simulink model "testifintegratoriscorrect"  (R2019a)
settings: Solver=FixedStepAuto  StartTime=0.0  StopTime=100  FixedStep=1e-4  RelTol=1e-5
InitFcn:
  | HeightAboveSeaLevel = 400 * rand;
  | Temperature = 288.15 + 30 * (rand - 0.5);
  | Pressure = 	101325 + 6000 * (rand - 0.5);
  | 
  | GustStart = 5 * rand;
  | GustLength = [100 + 50 * (rand - 0.5), 100 + 50 * (rand - 0.5), 100 + 50 * (rand - 0.5)];
  | GuestAmplitude = [ 10 * (rand - 0.5), 10 * (rand - 0.5),  10 * (rand - 0.5)];
  | 
  | ShearSpeed = 20 * rand;
  | ShearDirection = 360 * rand;
  | 
  | HeightAboveSeaLevel = 5.4419142084;
  | Temperature = 288.15;
  | Pressure = 	101325;
  | 
  | GustStart = 2.5;
  | GustLength = [100, 100, 100];
  | GuestAmplitude = [ 2.5, -2.5,  1];
  | 
  | ShearSpeed = 10;
  | ShearDirection = 180;
values from neighbouring files (symbols this model uses):
  D = zeros(size(B))    [RocketOutputFunction.m]    (also in StateSpaceController.m = zeros(13, 3); TimeDelayCompensationElevator.m = [0; 0])
  F = eye(6)    [MEKFAttitudeOnly.m]
  Ki2 = lqr(Ai2, Bi2, Q, R)    [StateSpaceController.m]
  q = x(13:16)    [AdaptiveLQR.m]    (also in MEKF.m = nominal_state(4:7); MEKFAttitudeOnly.m = [1 0 0 0]; MEKF_old.m = nominal_state(4:7); NonlinearStateEstimationForActuatorDelay.m = x(4:7))
  r = sym('r', [3 1])    [StateSpaceController.m]    (also in TimeDelayCompensationElevator.m = [0;0]; Tracker.m = [0; 0; -(rocket_length - Average_cg)])
  s = linspace(0, 100, nums)    [ImpactVelocityFunction.m]    (also in ImpactVelocityNotParallelMatlab.m = 1:5:500; ParallelImpactVelocity.m = .1:.01:500; ParralelRun.m = linspace(5,7, nums); RunImpactVelocityParforCompiled.m = 1:0.1:500)
undefined symbols (not defined in the file or in its folder): deg, e0_0, e1_0, e2_0, e3_0, Earth, Light, magnitude, MIL, rad, WGS84
libraries: aerolibutil x10, simulink x9, aerolibconvert2 x7, sharedtransform x7, shared6dof x7, aerolibwind2 x3, sharedutil x3, aerolibfltsims x2, aerolibasang x2, shared6dofsys x2, aerolibatmos2 x1, aerolibbdyn x1
(part 1 of 2)
settings Model: Creator=rag  LastModifiedBy=rag
settings SolverCC: ZeroCrossAlgorithm=Adaptive  MinimalZcImpactIntegration=on
settings DataIOCC: SaveOutput=off  SignalLogging=off  DSMLogging=off  SaveTime=off
settings DebuggingCC: ReadBeforeWriteMsg=DisableAll  WriteAfterWriteMsg=DisableAll  WriteAfterReadMsg=DisableAll  IgnoredZcDiagnostic=none  MultiTaskDSMMsg=none
settings ModelReferenceCC: UpdateModelReferenceTargets=IfOutOfDate
settings SFSimCC: SFSimEcho=off

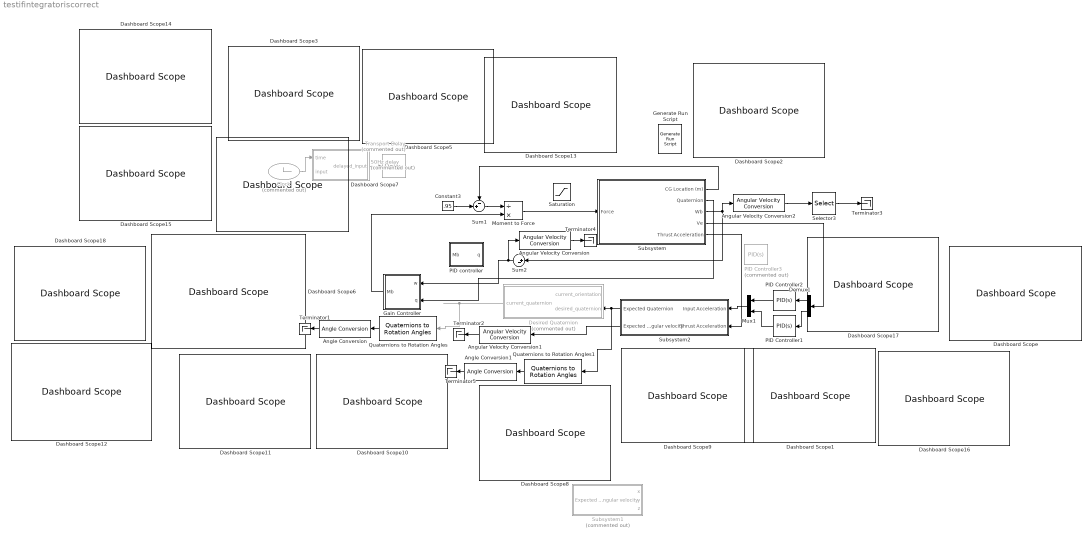
== system testifintegratoriscorrect ==
  50Hz delay : MATLAB Function  Commented=on  TreatAsAtomicUnit=on
  Angle Conversion : aerolibconvert2/Angle Conversion  IU=rad  OU=deg
  Angle Conversion1 : aerolibconvert2/Angle Conversion  IU=rad  OU=deg
  Angular Velocity Conversion : aerolibconvert2/Angular Velocity Conversion  IU=rad/s  OU=deg/s
      settings: SourceProductName=Aerospace Blockset
  Angular Velocity Conversion1 : aerolibconvert2/Angular Velocity Conversion  IU=rad/s  OU=deg/s
      settings: SourceProductName=Aerospace Blockset
  Angular Velocity Conversion2 : aerolibconvert2/Angular Velocity Conversion  IU=rad/s  OU=deg/s
      settings: SourceProductName=Aerospace Blockset
  Clock : Clock  Commented=on
      settings: Decimation=100
  Constant3 : Constant  Value=.95
  Dashboard Scope{,1..3,5..11,13..18} (17 alike) : DashboardScope
  Dashboard Scope12 : DashboardScope  Ymin=-1  Ymax=1
  Demux1 : Demux  Outputs=2
  Desired Quaternion : MATLAB Function  Commented=on  TreatAsAtomicUnit=on
  Gain Controller : Subsystem
  Generate Run Script : aerolibfltsims/Generate Run Script  Architecture=Win64  dataFlow=Send  GeometryModelName=Rocket  AirportId=PHNL  RunwayId=04L  InitialAltitude=13  InitialHeading=52.84  OffsetDistance=0  OffsetAzimuth=0  InstallScenery=off  DisableShaders=off  OriginAddress=127.0.0.1  DestinationPort=5502  OriginPort=5505  LocalAddress=127.0.0.1  OutputFileName=runfg.bat  FlightGearBaseDirectory=C:\Program Files\FlightGear 2018.2.2
  Moment to Force : Product  Inputs=/*
  Mux1 : Mux  Inputs=2
  PID Controller1 : simulink/Continuous/PID Controller  Controller=PID  Form=Parallel  TimeDomain=Continuous-time  SampleTime=-1  IntegratorMethod=Forward Euler  FilterMethod=Forward Euler  ControllerParametersSource=internal  P=-.5  I=-.5  D=0  UseFilter=on  N=10000  TunerSelectOption=Transfer Function Based (PID Tuner App)  InitialConditionSource=internal  InitialConditionForIntegrator=0  InitialConditionForFilter=0  DifferentiatorICPrevScaledInput=0  ExternalReset=none  TrackingMode=off  Kt=1  LimitOutput=off  UpperSaturationLimit=inf  LowerSaturationLimit=-inf  LinearizeAsGain=on  AntiWindupMode=none  Kb=1  POutMin=[]  POutMax=[]  IOutMin=[]  IOutMax=[]  DOutMin=[]  DOutMax=[]  NOutMin=[]  NOutMax=[]  SumOutMin=[]  SumOutMax=[]  SaturationOutMin=[]  SaturationOutMax=[]  PParamMin=[]  PParamMax=[]  IParamMin=[]  IParamMax=[]  DParamMin=[]  DParamMax=[]  NParamMin=[]  NParamMax=[]  KbParamMin=[]  KbParamMax=[]  KtParamMin=[]  KtParamMax=[]  KbOutMin=[]  KbOutMax=[]  KtOutMin=[]  KtOutMax=[]  IntegratorOutMin=[]  IntegratorOutMax=[]  FilterOutMin=[]  FilterOutMax=[]  SumI1OutMin=[]  SumI1OutMax=[]  SumI2OutMin=[]  SumI2OutMax=[]  SumI3OutMin=[]  SumI3OutMax=[]  SumI4OutMin=[]  SumI4OutMax=[]  SumDOutMin=[]  SumDOutMax=[]  DifferentiatorOutMin=[]  DifferentiatorOutMax=[]  FilterDiffOutCoefMin=[]  FilterDiffOutCoefMax=[]  ReciprocalOutMin=[]  ReciprocalOutMax=[]  SumDenOutMin=[]  SumDenOutMax=[]  SumNumOutMin=[]  SumNumOutMax=[]  DivideOutMin=[]  DivideOutMax=[]  IntegratorContinuousStateAttributes=''  IntegratorStateMustResolveToSignalObject=off  IntegratorRTWStateStorageClass=Auto  FilterContinuousStateAttributes=''  FilterStateMustResolveToSignalObject=off  FilterRTWStateStorageClass=Auto  ParallelPVariant=InternalParameters  IdealPVariant=Disabled  IVariant=InternalParameters  DVariant=InternalParameters  IntegratorVariant=Continuous  SatVariant=Disabled  AWVariant=Passthrough  PCopyVariant=Disabled  TRVariant=Disabled  FdbkBlocksVariant=Forward  IdealPFdbkVariant=Disabled  SatFdbkVariant=Disabled  DerivativeFilterVariant=ContFilter  NVariant=InternalParameters  NCopyVariant=Disabled  FilterICVariant=InternalICsFilter  IntegratorICVariant=InternalICs  ExternalResetVariant=Disabled  TRSumVariant=Passthrough  SumFdbkVariant=Disabled  SumVariant=Sum_PID
  PID Controller2 : simulink/Continuous/PID Controller  Controller=PID  Form=Parallel  TimeDomain=Continuous-time  SampleTime=-1  IntegratorMethod=Forward Euler  FilterMethod=Forward Euler  ControllerParametersSource=internal  P=-.5  I=-.5  D=0  UseFilter=on  N=10000  TunerSelectOption=Transfer Function Based (PID Tuner App)  InitialConditionSource=internal  InitialConditionForIntegrator=0  InitialConditionForFilter=0  DifferentiatorICPrevScaledInput=0  ExternalReset=none  TrackingMode=off  Kt=1  LimitOutput=off  UpperSaturationLimit=inf  LowerSaturationLimit=-inf  LinearizeAsGain=on  AntiWindupMode=none  Kb=1  POutMin=[]  POutMax=[]  IOutMin=[]  IOutMax=[]  DOutMin=[]  DOutMax=[]  NOutMin=[]  NOutMax=[]  SumOutMin=[]  SumOutMax=[]  SaturationOutMin=[]  SaturationOutMax=[]  PParamMin=[]  PParamMax=[]  IParamMin=[]  IParamMax=[]  DParamMin=[]  DParamMax=[]  NParamMin=[]  NParamMax=[]  KbParamMin=[]  KbParamMax=[]  KtParamMin=[]  KtParamMax=[]  KbOutMin=[]  KbOutMax=[]  KtOutMin=[]  KtOutMax=[]  IntegratorOutMin=[]  IntegratorOutMax=[]  FilterOutMin=[]  FilterOutMax=[]  SumI1OutMin=[]  SumI1OutMax=[]  SumI2OutMin=[]  SumI2OutMax=[]  SumI3OutMin=[]  SumI3OutMax=[]  SumI4OutMin=[]  SumI4OutMax=[]  SumDOutMin=[]  SumDOutMax=[]  DifferentiatorOutMin=[]  DifferentiatorOutMax=[]  FilterDiffOutCoefMin=[]  FilterDiffOutCoefMax=[]  ReciprocalOutMin=[]  ReciprocalOutMax=[]  SumDenOutMin=[]  SumDenOutMax=[]  SumNumOutMin=[]  SumNumOutMax=[]  DivideOutMin=[]  DivideOutMax=[]  IntegratorContinuousStateAttributes=''  IntegratorStateMustResolveToSignalObject=off  IntegratorRTWStateStorageClass=Auto  FilterContinuousStateAttributes=''  FilterStateMustResolveToSignalObject=off  FilterRTWStateStorageClass=Auto  ParallelPVariant=InternalParameters  IdealPVariant=Disabled  IVariant=InternalParameters  DVariant=InternalParameters  IntegratorVariant=Continuous  SatVariant=Disabled  AWVariant=Passthrough  PCopyVariant=Disabled  TRVariant=Disabled  FdbkBlocksVariant=Forward  IdealPFdbkVariant=Disabled  SatFdbkVariant=Disabled  DerivativeFilterVariant=ContFilter  NVariant=InternalParameters  NCopyVariant=Disabled  FilterICVariant=InternalICsFilter  IntegratorICVariant=InternalICs  ExternalResetVariant=Disabled  TRSumVariant=Passthrough  SumFdbkVariant=Disabled  SumVariant=Sum_PID
  PID Controller3 : simulink/Continuous/PID Controller  Commented=on  Controller=PID  Form=Parallel  TimeDomain=Continuous-time  SampleTime=-1  IntegratorMethod=Forward Euler  FilterMethod=Forward Euler  ControllerParametersSource=internal  P=-0.123834085166626  I=-0.0589771468563032  D=0.0137648749687481  UseFilter=on  N=8.99638285475018  TunerSelectOption=Transfer Function Based (PID Tuner App)  InitialConditionSource=internal  InitialConditionForIntegrator=0  InitialConditionForFilter=0  DifferentiatorICPrevScaledInput=0  ExternalReset=none  TrackingMode=off  Kt=1  LimitOutput=off  UpperSaturationLimit=inf  LowerSaturationLimit=-inf  LinearizeAsGain=on  AntiWindupMode=none  Kb=1  POutMin=[]  POutMax=[]  IOutMin=[]  IOutMax=[]  DOutMin=[]  DOutMax=[]  NOutMin=[]  NOutMax=[]  SumOutMin=[]  SumOutMax=[]  SaturationOutMin=[]  SaturationOutMax=[]  PParamMin=[]  PParamMax=[]  IParamMin=[]  IParamMax=[]  DParamMin=[]  DParamMax=[]  NParamMin=[]  NParamMax=[]  KbParamMin=[]  KbParamMax=[]  KtParamMin=[]  KtParamMax=[]  KbOutMin=[]  KbOutMax=[]  KtOutMin=[]  KtOutMax=[]  IntegratorOutMin=[]  IntegratorOutMax=[]  FilterOutMin=[]  FilterOutMax=[]  SumI1OutMin=[]  SumI1OutMax=[]  SumI2OutMin=[]  SumI2OutMax=[]  SumI3OutMin=[]  SumI3OutMax=[]  SumI4OutMin=[]  SumI4OutMax=[]  SumDOutMin=[]  SumDOutMax=[]  DifferentiatorOutMin=[]  DifferentiatorOutMax=[]  FilterDiffOutCoefMin=[]  FilterDiffOutCoefMax=[]  ReciprocalOutMin=[]  ReciprocalOutMax=[]  SumDenOutMin=[]  SumDenOutMax=[]  SumNumOutMin=[]  SumNumOutMax=[]  DivideOutMin=[]  DivideOutMax=[]  IntegratorContinuousStateAttributes=''  IntegratorStateMustResolveToSignalObject=off  IntegratorRTWStateStorageClass=Auto  FilterContinuousStateAttributes=''  FilterStateMustResolveToSignalObject=off  FilterRTWStateStorageClass=Auto  ParallelPVariant=InternalParameters  IdealPVariant=Disabled  IVariant=InternalParameters  DVariant=InternalParameters  IntegratorVariant=Continuous  SatVariant=Disabled  AWVariant=Passthrough  PCopyVariant=Disabled  TRVariant=Disabled  FdbkBlocksVariant=Forward  IdealPFdbkVariant=Disabled  SatFdbkVariant=Disabled  DerivativeFilterVariant=ContFilter  NVariant=InternalParameters  NCopyVariant=Disabled  FilterICVariant=InternalICsFilter  IntegratorICVariant=InternalICs  ExternalResetVariant=Disabled  TRSumVariant=Passthrough  SumFdbkVariant=Disabled  SumVariant=Sum_PID
  PID controller : Subsystem
  Quaternions to Rotation Angles : sharedtransform/Quaternions to Rotation Angles  rotationOrder=ZYX  aMode=aMode
      settings: SourceProductBaseCode=AE
  Quaternions to Rotation Angles1 : sharedtransform/Quaternions to Rotation Angles  rotationOrder=XYZ  aMode=aMode
      settings: SourceProductBaseCode=AE
  Saturation : Saturate  UpperLimit=1.5  LowerLimit=-1.5
  Selector3 : Selector  InputPortWidth=3  IndexOptions=Index vector (dialog)  Indices=[1 2]  OutputSizes=1
  Subsystem : Subsystem
  Subsystem1 : Subsystem  Commented=on
  Subsystem2 : Subsystem
  Sum1 : Sum  Inputs=-+|
  Sum2 : Sum  Inputs=|+-
  Terminator{1..5} (5 alike) : Terminator
  Transport Delay : TransportDelay  Commented=on  DelayTime=0.015  TransDelayFeedthrough=on
  wires:
  Subsystem/3(Wb) -> Sum2/1, Angular Velocity Conversion2/1
  Clock/1 -> 50Hz delay/1(time)
  50Hz delay/1(delayed_input) -> Transport Delay/1
  Sum2/1 -> Gain Controller/1(w), Angular Velocity Conversion/1
  Subsystem/5(Thrust Acceleration) -> Subsystem2/2(Thrust Acceleration)
  Angular Velocity Conversion1/1 -> Terminator2/1
  Subsystem2/2(Expected angular velocity) -> Angular Velocity Conversion1/1
  Quaternions to Rotation Angles/1 -> Angle Conversion/1
  Subsystem/1(CG Location (m)) -> Sum1/1
  Sum1/1 -> Moment to Force/1
  Constant3/1 -> Sum1/2
  Angle Conversion/1 -> Terminator1/1
  Angular Velocity Conversion2/1 -> Selector3/1
  Angular Velocity Conversion/1 -> Terminator4/1
  Angle Conversion1/1 -> Terminator5/1
  Subsystem2/1(Expected Quaternion) -> Desired Quaternion/2(desired_quaternion), Quaternions to Rotation Angles1/1
  Quaternions to Rotation Angles1/1 -> Angle Conversion1/1
  Desired Quaternion/1(current_quaternion) -> Quaternions to Rotation Angles/1
  Subsystem/2(Quaternion) -> Gain Controller/2(q)
  Gain Controller/1(Mb) -> Moment to Force/2
  Moment to Force/1 -> Subsystem/1(Force)
  Selector3/1 -> Terminator3/1
  Demux1/1 -> PID Controller2/1
  Mux1/1 -> Subsystem2/1(Input Acceleration)
  PID Controller2/1 -> Mux1/1
  Subsystem/4(Ve) -> Demux1/1
  Demux1/2 -> PID Controller1/1
  PID Controller1/1 -> Mux1/2

== system testifintegratoriscorrect/Gain Controller ==
  w : Inport
  q : Inport  Port=2
  Derivative : Derivative
  Gain : Gain  Gain=-Ki2  Multiplication=Matrix(K*u)
  Integrator : Integrator
  Reshape1 : Reshape  OutputDimensionality=Column vector (2-D)
  Selector1 : Selector  InputPortWidth=3  IndexOptions=Index vector (dialog)  Indices=[2 1]  OutputSizes=1
  Selector2 : Selector  InputPortWidth=4  IndexOptions=Index vector (dialog)  Indices=[3 2]  OutputSizes=1
  Vector Concatenate4 : Concatenate  NumInputs=3
  Mb : Outport
  wires:
  Vector Concatenate4/1 -> Reshape1/1
  Reshape1/1 -> Gain/1
  Selector2/1 -> Derivative/1, Integrator/1, Vector Concatenate4/2
  Integrator/1 -> Vector Concatenate4/3
  q/1 -> Selector2/1
  Gain/1 -> Mb/1
  Selector1/1 -> Vector Concatenate4/1
  w/1 -> Selector1/1

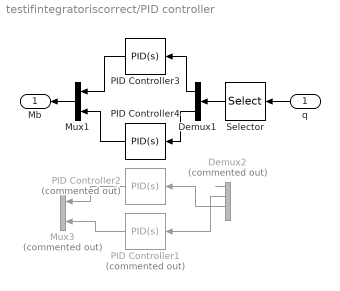
== system testifintegratoriscorrect/PID controller ==
  q : Inport
  Demux1 : Demux  Outputs=2
  Demux2 : Demux  Commented=on
  Mux1 : Mux  Inputs=2
  Mux3 : Mux  Commented=on  Inputs=2
  PID Controller1 : simulink/Continuous/PID Controller  Commented=on  Controller=PID  Form=Parallel  TimeDomain=Continuous-time  SampleTime=-1  IntegratorMethod=Forward Euler  FilterMethod=Forward Euler  ControllerParametersSource=internal  P=-19.0768820466686  I=-17.6802234864968  D=-5.0952523858048  UseFilter=on  N=209.794311620465  TunerSelectOption=Transfer Function Based (PID Tuner App)  InitialConditionSource=internal  InitialConditionForIntegrator=0  InitialConditionForFilter=0  DifferentiatorICPrevScaledInput=0  ExternalReset=none  TrackingMode=off  Kt=1  LimitOutput=off  UpperSaturationLimit=inf  LowerSaturationLimit=-inf  LinearizeAsGain=on  AntiWindupMode=none  Kb=1  POutMin=[]  POutMax=[]  IOutMin=[]  IOutMax=[]  DOutMin=[]  DOutMax=[]  NOutMin=[]  NOutMax=[]  SumOutMin=[]  SumOutMax=[]  SaturationOutMin=[]  SaturationOutMax=[]  PParamMin=[]  PParamMax=[]  IParamMin=[]  IParamMax=[]  DParamMin=[]  DParamMax=[]  NParamMin=[]  NParamMax=[]  KbParamMin=[]  KbParamMax=[]  KtParamMin=[]  KtParamMax=[]  KbOutMin=[]  KbOutMax=[]  KtOutMin=[]  KtOutMax=[]  IntegratorOutMin=[]  IntegratorOutMax=[]  FilterOutMin=[]  FilterOutMax=[]  SumI1OutMin=[]  SumI1OutMax=[]  SumI2OutMin=[]  SumI2OutMax=[]  SumI3OutMin=[]  SumI3OutMax=[]  SumI4OutMin=[]  SumI4OutMax=[]  SumDOutMin=[]  SumDOutMax=[]  DifferentiatorOutMin=[]  DifferentiatorOutMax=[]  FilterDiffOutCoefMin=[]  FilterDiffOutCoefMax=[]  ReciprocalOutMin=[]  ReciprocalOutMax=[]  SumDenOutMin=[]  SumDenOutMax=[]  SumNumOutMin=[]  SumNumOutMax=[]  DivideOutMin=[]  DivideOutMax=[]  IntegratorContinuousStateAttributes=''  IntegratorStateMustResolveToSignalObject=off  IntegratorRTWStateStorageClass=Auto  FilterContinuousStateAttributes=''  FilterStateMustResolveToSignalObject=off  FilterRTWStateStorageClass=Auto  ParallelPVariant=InternalParameters  IdealPVariant=Disabled  IVariant=InternalParameters  DVariant=InternalParameters  IntegratorVariant=Continuous  SatVariant=Disabled  AWVariant=Passthrough  PCopyVariant=Disabled  TRVariant=Disabled  FdbkBlocksVariant=Forward  IdealPFdbkVariant=Disabled  SatFdbkVariant=Disabled  DerivativeFilterVariant=ContFilter  NVariant=InternalParameters  NCopyVariant=Disabled  FilterICVariant=InternalICsFilter  IntegratorICVariant=InternalICs  ExternalResetVariant=Disabled  TRSumVariant=Passthrough  SumFdbkVariant=Disabled  SumVariant=Sum_PID
  PID Controller2 : simulink/Continuous/PID Controller  Commented=on  Controller=PID  Form=Parallel  TimeDomain=Continuous-time  SampleTime=-1  IntegratorMethod=Forward Euler  FilterMethod=Forward Euler  ControllerParametersSource=internal  P=-19.0768820466686  I=-17.6802234864968  D=-5.0952523858048  UseFilter=on  N=209.794311620465  TunerSelectOption=Transfer Function Based (PID Tuner App)  InitialConditionSource=internal  InitialConditionForIntegrator=0  InitialConditionForFilter=0  DifferentiatorICPrevScaledInput=0  ExternalReset=none  TrackingMode=off  Kt=1  LimitOutput=off  UpperSaturationLimit=inf  LowerSaturationLimit=-inf  LinearizeAsGain=on  AntiWindupMode=none  Kb=1  POutMin=[]  POutMax=[]  IOutMin=[]  IOutMax=[]  DOutMin=[]  DOutMax=[]  NOutMin=[]  NOutMax=[]  SumOutMin=[]  SumOutMax=[]  SaturationOutMin=[]  SaturationOutMax=[]  PParamMin=[]  PParamMax=[]  IParamMin=[]  IParamMax=[]  DParamMin=[]  DParamMax=[]  NParamMin=[]  NParamMax=[]  KbParamMin=[]  KbParamMax=[]  KtParamMin=[]  KtParamMax=[]  KbOutMin=[]  KbOutMax=[]  KtOutMin=[]  KtOutMax=[]  IntegratorOutMin=[]  IntegratorOutMax=[]  FilterOutMin=[]  FilterOutMax=[]  SumI1OutMin=[]  SumI1OutMax=[]  SumI2OutMin=[]  SumI2OutMax=[]  SumI3OutMin=[]  SumI3OutMax=[]  SumI4OutMin=[]  SumI4OutMax=[]  SumDOutMin=[]  SumDOutMax=[]  DifferentiatorOutMin=[]  DifferentiatorOutMax=[]  FilterDiffOutCoefMin=[]  FilterDiffOutCoefMax=[]  ReciprocalOutMin=[]  ReciprocalOutMax=[]  SumDenOutMin=[]  SumDenOutMax=[]  SumNumOutMin=[]  SumNumOutMax=[]  DivideOutMin=[]  DivideOutMax=[]  IntegratorContinuousStateAttributes=''  IntegratorStateMustResolveToSignalObject=off  IntegratorRTWStateStorageClass=Auto  FilterContinuousStateAttributes=''  FilterStateMustResolveToSignalObject=off  FilterRTWStateStorageClass=Auto  ParallelPVariant=InternalParameters  IdealPVariant=Disabled  IVariant=InternalParameters  DVariant=InternalParameters  IntegratorVariant=Continuous  SatVariant=Disabled  AWVariant=Passthrough  PCopyVariant=Disabled  TRVariant=Disabled  FdbkBlocksVariant=Forward  IdealPFdbkVariant=Disabled  SatFdbkVariant=Disabled  DerivativeFilterVariant=ContFilter  NVariant=InternalParameters  NCopyVariant=Disabled  FilterICVariant=InternalICsFilter  IntegratorICVariant=InternalICs  ExternalResetVariant=Disabled  TRSumVariant=Passthrough  SumFdbkVariant=Disabled  SumVariant=Sum_PID
  PID Controller3 : simulink/Continuous/PID Controller  Controller=PID  Form=Parallel  TimeDomain=Continuous-time  SampleTime=-1  IntegratorMethod=Forward Euler  FilterMethod=Forward Euler  ControllerParametersSource=internal  P=-19.0768820466686  I=-17.6802234864968  D=-5.0952523858048  UseFilter=on  N=209.794311620465  TunerSelectOption=Transfer Function Based (PID Tuner App)  InitialConditionSource=internal  InitialConditionForIntegrator=0  InitialConditionForFilter=0  DifferentiatorICPrevScaledInput=0  ExternalReset=none  TrackingMode=off  Kt=1  LimitOutput=off  UpperSaturationLimit=inf  LowerSaturationLimit=-inf  LinearizeAsGain=on  AntiWindupMode=none  Kb=1  POutMin=[]  POutMax=[]  IOutMin=[]  IOutMax=[]  DOutMin=[]  DOutMax=[]  NOutMin=[]  NOutMax=[]  SumOutMin=[]  SumOutMax=[]  SaturationOutMin=[]  SaturationOutMax=[]  PParamMin=[]  PParamMax=[]  IParamMin=[]  IParamMax=[]  DParamMin=[]  DParamMax=[]  NParamMin=[]  NParamMax=[]  KbParamMin=[]  KbParamMax=[]  KtParamMin=[]  KtParamMax=[]  KbOutMin=[]  KbOutMax=[]  KtOutMin=[]  KtOutMax=[]  IntegratorOutMin=[]  IntegratorOutMax=[]  FilterOutMin=[]  FilterOutMax=[]  SumI1OutMin=[]  SumI1OutMax=[]  SumI2OutMin=[]  SumI2OutMax=[]  SumI3OutMin=[]  SumI3OutMax=[]  SumI4OutMin=[]  SumI4OutMax=[]  SumDOutMin=[]  SumDOutMax=[]  DifferentiatorOutMin=[]  DifferentiatorOutMax=[]  FilterDiffOutCoefMin=[]  FilterDiffOutCoefMax=[]  ReciprocalOutMin=[]  ReciprocalOutMax=[]  SumDenOutMin=[]  SumDenOutMax=[]  SumNumOutMin=[]  SumNumOutMax=[]  DivideOutMin=[]  DivideOutMax=[]  IntegratorContinuousStateAttributes=''  IntegratorStateMustResolveToSignalObject=off  IntegratorRTWStateStorageClass=Auto  FilterContinuousStateAttributes=''  FilterStateMustResolveToSignalObject=off  FilterRTWStateStorageClass=Auto  ParallelPVariant=InternalParameters  IdealPVariant=Disabled  IVariant=InternalParameters  DVariant=InternalParameters  IntegratorVariant=Continuous  SatVariant=Disabled  AWVariant=Passthrough  PCopyVariant=Disabled  TRVariant=Disabled  FdbkBlocksVariant=Forward  IdealPFdbkVariant=Disabled  SatFdbkVariant=Disabled  DerivativeFilterVariant=ContFilter  NVariant=InternalParameters  NCopyVariant=Disabled  FilterICVariant=InternalICsFilter  IntegratorICVariant=InternalICs  ExternalResetVariant=Disabled  TRSumVariant=Passthrough  SumFdbkVariant=Disabled  SumVariant=Sum_PID
  PID Controller4 : simulink/Continuous/PID Controller  Controller=PID  Form=Parallel  TimeDomain=Continuous-time  SampleTime=-1  IntegratorMethod=Forward Euler  FilterMethod=Forward Euler  ControllerParametersSource=internal  P=-19.0768820466686  I=-17.6802234864968  D=-5.0952523858048  UseFilter=on  N=209.794311620465  TunerSelectOption=Transfer Function Based (PID Tuner App)  InitialConditionSource=internal  InitialConditionForIntegrator=0  InitialConditionForFilter=0  DifferentiatorICPrevScaledInput=0  ExternalReset=none  TrackingMode=off  Kt=1  LimitOutput=off  UpperSaturationLimit=inf  LowerSaturationLimit=-inf  LinearizeAsGain=on  AntiWindupMode=none  Kb=1  POutMin=[]  POutMax=[]  IOutMin=[]  IOutMax=[]  DOutMin=[]  DOutMax=[]  NOutMin=[]  NOutMax=[]  SumOutMin=[]  SumOutMax=[]  SaturationOutMin=[]  SaturationOutMax=[]  PParamMin=[]  PParamMax=[]  IParamMin=[]  IParamMax=[]  DParamMin=[]  DParamMax=[]  NParamMin=[]  NParamMax=[]  KbParamMin=[]  KbParamMax=[]  KtParamMin=[]  KtParamMax=[]  KbOutMin=[]  KbOutMax=[]  KtOutMin=[]  KtOutMax=[]  IntegratorOutMin=[]  IntegratorOutMax=[]  FilterOutMin=[]  FilterOutMax=[]  SumI1OutMin=[]  SumI1OutMax=[]  SumI2OutMin=[]  SumI2OutMax=[]  SumI3OutMin=[]  SumI3OutMax=[]  SumI4OutMin=[]  SumI4OutMax=[]  SumDOutMin=[]  SumDOutMax=[]  DifferentiatorOutMin=[]  DifferentiatorOutMax=[]  FilterDiffOutCoefMin=[]  FilterDiffOutCoefMax=[]  ReciprocalOutMin=[]  ReciprocalOutMax=[]  SumDenOutMin=[]  SumDenOutMax=[]  SumNumOutMin=[]  SumNumOutMax=[]  DivideOutMin=[]  DivideOutMax=[]  IntegratorContinuousStateAttributes=''  IntegratorStateMustResolveToSignalObject=off  IntegratorRTWStateStorageClass=Auto  FilterContinuousStateAttributes=''  FilterStateMustResolveToSignalObject=off  FilterRTWStateStorageClass=Auto  ParallelPVariant=InternalParameters  IdealPVariant=Disabled  IVariant=InternalParameters  DVariant=InternalParameters  IntegratorVariant=Continuous  SatVariant=Disabled  AWVariant=Passthrough  PCopyVariant=Disabled  TRVariant=Disabled  FdbkBlocksVariant=Forward  IdealPFdbkVariant=Disabled  SatFdbkVariant=Disabled  DerivativeFilterVariant=ContFilter  NVariant=InternalParameters  NCopyVariant=Disabled  FilterICVariant=InternalICsFilter  IntegratorICVariant=InternalICs  ExternalResetVariant=Disabled  TRSumVariant=Passthrough  SumFdbkVariant=Disabled  SumVariant=Sum_PID
  Selector : Selector  InputPortWidth=4  IndexOptions=Index vector (dialog)  Indices=[3 2]  OutputSizes=1
  Mb : Outport
  wires:
  q/1 -> Selector/1
  PID Controller1/1 -> Mux3/2
  Demux2/3 -> PID Controller2/1
  PID Controller2/1 -> Mux3/1
  Demux2/2 -> PID Controller1/1
  Demux2/1 -> ?
  Selector/1 -> Demux1/1
  PID Controller3/1 -> Mux1/1
  Demux1/1 -> PID Controller3/1
  Demux1/2 -> PID Controller4/1
  PID Controller4/1 -> Mux1/2
  Mux1/1 -> Mb/1

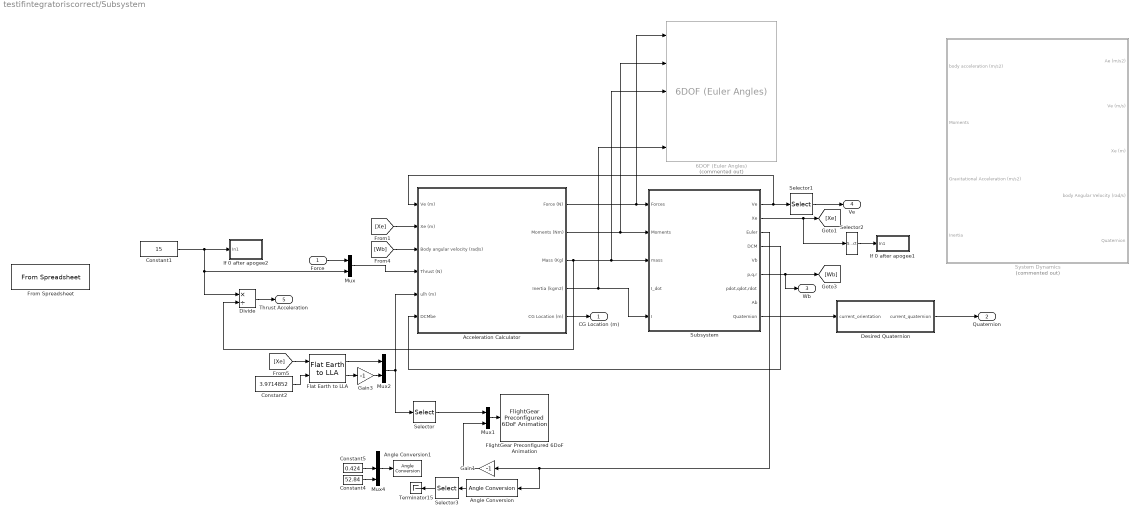
== system testifintegratoriscorrect/Subsystem ==
  Force : Inport  PortDimensions=2
  6DOF (Euler Angles) : shared6dof/6DOF (Euler Angles)  Commented=on  units=Metric (MKS)  mtype=Custom Variable  rep=Quaternion  xme_0=[0 0 0]  Vm_0=[0 0 0]  eul_0=[0 0 0]  pm_0=[0 0 0]  mass_0=1.0  mass_e=0.5  mass_f=2.0  inertia=eye(3)  inertia_e=eye(3)  inertia_f=2*eye(3)  k_quat=1.0  vre_flag=off  abi_flag=off  aMode=0  xme_statename=''  Vm_statename=''  eul_statename=''  quat_statename=''  pm_statename=''  mass_statename=''
      settings: SourceProductBaseCode=AE
  Acceleration Calculator : Subsystem
  Angle Conversion : aerolibconvert2/Angle Conversion  IU=rad  OU=deg
  Angle Conversion1 : aerolibconvert2/Angle Conversion  IU=deg  OU=rad
  Constant1 : Constant  Value=15
  Constant2 : Constant  Value=3.9714852
  Constant4 : Constant  Value=52.84
  Constant5 : Constant  Value=0.424
  Desired Quaternion : MATLAB Function  TreatAsAtomicUnit=on
  Divide : Product  Inputs=*/
  Flat Earth to LLA : aerolibtransform2/Flat Earth to LLA  units=Metric (MKS)  ptype=Earth (WGS84)  F=1/298.257223563  R=6378137  LL0=[21.318358277648 -157.9232805920725]  psi=0
  FlightGear Preconfigured 6DoF Animation : aerolibfltsims/FlightGear Preconfigured 6DoF Animation  xFlightGearVersion=v2018.2  DestinationIpAddress=127.0.0.1  DestinationPort=5502  SampleTime=1/50  packetVersion=24
      settings: SourceProductName=Aerospace Blockset
  From Spreadsheet : FromSpreadsheet  FileName=F10_Thrust.xls  Range=A1:B29  ExtrapolationBeforeFirstDataPoint=Hold first value  ExtrapolationAfterLastDataPoint=Hold last value
  Gain1 : Gain  Gain=-1
  Gain3 : Gain  Gain=-1
  If 0 after apogee1 : Subsystem
  If 0 after apogee2 : Subsystem
  Mux : Mux  Inputs=2
  Mux1 : Mux  Inputs=2
  Mux2 : Mux  Inputs=2
  Mux4 : Mux  Inputs=3
  Selector : Selector  InputPortWidth=3  IndexOptions=Index vector (dialog)  Indices=[2 1 3]  OutputSizes=1
  Selector1 : Selector  InputPortWidth=3  IndexOptions=Index vector (dialog)  Indices=[1 2]  OutputSizes=1
  Selector2 : Selector  InputPortWidth=3  IndexOptions=Index vector (dialog)  Indices=[3]  OutputSizes=1
  Selector3 : Selector  InputPortWidth=3  IndexOptions=Index vector (dialog)  Indices=[1 2]  OutputSizes=1
  Subsystem : Subsystem
  System Dynamics : Subsystem  Commented=on
  Terminator15 : Terminator
  CG Location (m) : Outport
  Quaternion : Outport  Port=2
  Wb : Outport  Port=3
  Ve : Outport  Port=4
  Thrust Acceleration : Outport  Port=5
  wires:
  Selector/1 -> Mux1/1
  Flat Earth to LLA/1 -> Mux2/1
  Flat Earth to LLA/2 -> Gain3/1
  Gain3/1 -> Mux2/2
  Mux2/1 -> Acceleration Calculator/5(ulh (m)), Selector/1
  Constant2/1 -> Flat Earth to LLA/2
  Subsystem/1(Ve) -> Acceleration Calculator/1(Ve (m)), Selector1/1
  Mux1/1 -> FlightGear Preconfigured 6DoF Animation/1
  [Xe] -> Acceleration Calculator/2(Xe (m))
  Force/1 -> Mux/1
  Selector2/1 -> If 0 after apogee1/1(In1)
  Constant4/1 -> Mux4/3
  Mux4/1 -> Angle Conversion1/1
  Constant5/1 -> Mux4/2
  [Xe] -> Flat Earth to LLA/1
  Divide/1 -> Thrust Acceleration/1
  [Wb] -> Acceleration Calculator/3(Body angular velocity (rad/s))
  Acceleration Calculator/5(CG Location (m)) -> CG Location (m)/1
  Selector1/1 -> Ve/1
  Angle Conversion/1 -> Selector3/1
  Acceleration Calculator/4(Inertia (kgm2)) -> 6DOF (Euler Angles)/5, Subsystem/5(I)
  Acceleration Calculator/2(Moments (Nm)) -> 6DOF (Euler Angles)/2, Subsystem/2(Moments)
  Acceleration Calculator/1(Force (N)) -> Subsystem/1(Forces), 6DOF (Euler Angles)/1
  Subsystem/2(Xe) -> Selector2/1, [Xe]
  Subsystem/4(DCM) -> Acceleration Calculator/6(DCMbe)
  Selector3/1 -> Terminator15/1
  Constant1/1 -> Divide/1, Mux/2, If 0 after apogee2/1(In1)
  Acceleration Calculator/3(Mass (Kg)) -> 6DOF (Euler Angles)/3, Subsystem/3(mass), Divide/2
  Subsystem/6(p,q,r) -> Wb/1, [Wb]
  Subsystem/9(Quaternion) -> Desired Quaternion/1(current_orientation)
  Desired Quaternion/1(current_quaternion) -> Quaternion/1
  Mux/1 -> Acceleration Calculator/4(Thrust (N))
  Subsystem/3(Euler) -> Angle Conversion/1, Gain1/1
  Gain1/1 -> Mux1/2

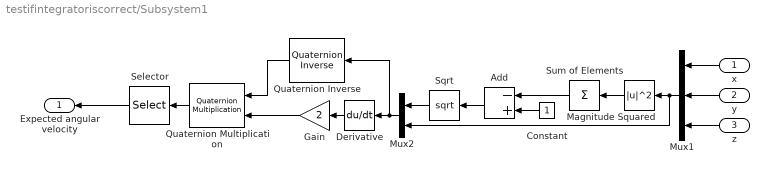
== system testifintegratoriscorrect/Subsystem1 ==
  x : Inport
  y : Inport  Port=2
  z : Inport  Port=3
  Add : Sum  Inputs=-+
  Constant : Constant
  Derivative : Derivative
  Gain : Gain  Gain=2
  Magnitude Squared : Math  Operator=magnitude^2  SaturateOnIntegerOverflow=on
  Mux1 : Mux  Inputs=3
  Mux2 : Mux  Inputs=2
  Quaternion Inverse : aerolibutil/Quaternion Inverse
      settings: SourceProductName=Aerospace Blockset
  Quaternion Multiplication : aerolibutil/Quaternion Multiplication
  Selector : Selector  InputPortWidth=4  IndexOptions=Index vector (dialog)  Indices=[2 3 4]  OutputSizes=1
  Sqrt : Sqrt  SaturateOnIntegerOverflow=on
  Sum of Elements : Sum  Inputs=+
  Expected angular velocity : Outport
  wires:
  Quaternion Inverse/1 -> Quaternion Multiplication/1
  x/1 -> Mux1/1
  Gain/1 -> Quaternion Multiplication/2
  Magnitude Squared/1 -> Sum of Elements/1
  Add/1 -> Sqrt/1
  Mux1/1 -> Mux2/2, Magnitude Squared/1
  Quaternion Multiplication/1 -> Selector/1
  Mux2/1 -> Quaternion Inverse/1, Derivative/1
  Constant/1 -> Add/2
  Derivative/1 -> Gain/1
  Sqrt/1 -> Mux2/1
  z/1 -> Mux1/3
  y/1 -> Mux1/2
  Sum of Elements/1 -> Add/1
  Selector/1 -> Expected angular velocity/1

== system testifintegratoriscorrect/Subsystem2 ==
  Input Acceleration : Inport  PortDimensions=[2]
  Thrust Acceleration : Inport  Port=2
  Derivative : Derivative
  Desired Quaternion : MATLAB Function  TreatAsAtomicUnit=on
  Gain : Gain  Gain=2
  Expected Quaternion : Outport
  Expected angular velocity : Outport  Port=2
  wires:
  Thrust Acceleration/1 -> Desired Quaternion/2(thrust_acceleration)
  Gain/1 -> Expected angular velocity/1
  Desired Quaternion/1(desired_quaternion) -> Expected Quaternion/1
  Input Acceleration/1 -> Desired Quaternion/1(input_acceleration)
  Derivative/1 -> Gain/1
  Desired Quaternion/2(ln_quat) -> Derivative/1

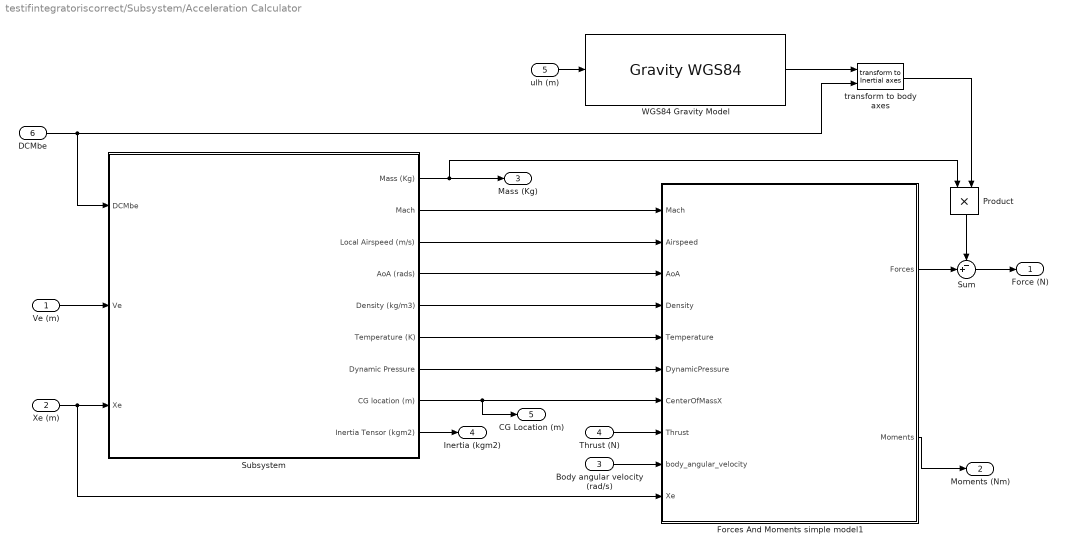
== system testifintegratoriscorrect/Subsystem/Acceleration Calculator ==
  Ve (m) : Inport
  Xe (m) : Inport  Port=2
  Body angular velocity (rad/s) : Inport  Port=3
  Thrust (N) : Inport  Port=4
  ulh (m) : Inport  Port=5
  DCMbe : Inport  Port=6
  Forces And Moments simple model1 : MATLAB Function  TreatAsAtomicUnit=on
  Product : Product
  Subsystem : Subsystem
  Sum : Sum  Inputs=-+|
  "WGS84 Gravity Model  " : GravityWGS84
  "transform to body axes " : shared6dof/6DOF (Euler Angles)/transform to Inertial axes   SystemSampleTime=-1
      settings: SourceProductName=Aerospace Blockset  SourceProductBaseCode=AE
  Force (N) : Outport
  Moments (Nm) : Outport  Port=2
  Mass (Kg) : Outport  Port=3
  Inertia (kgm2) : Outport  Port=4
  CG Location (m) : Outport  Port=5
  wires:
  Subsystem/4(AoA (rads)) -> Forces And Moments simple model1/3(AoA)
  Xe (m)/1 -> Forces And Moments simple model1/10(Xe), Subsystem/3(Xe)
  Subsystem/6(Temperature (K)) -> Forces And Moments simple model1/5(Temperature)
  Subsystem/8(CG location (m)) -> CG Location (m)/1, Forces And Moments simple model1/7(CenterOfMassX)
  Subsystem/3(Local Airspeed (m/s)) -> Forces And Moments simple model1/2(Airspeed)
  Subsystem/7(Dynamic Pressure) -> Forces And Moments simple model1/6(DynamicPressure)
  Subsystem/2(Mach) -> Forces And Moments simple model1/1(Mach)
  Subsystem/5(Density (kg/m3)) -> Forces And Moments simple model1/4(Density)
  Thrust (N)/1 -> Forces And Moments simple model1/8(Thrust)
  Body angular velocity (rad/s)/1 -> Forces And Moments simple model1/9(body_angular_velocity)
  Ve (m)/1 -> Subsystem/2(Ve)
  Subsystem/9(Inertia Tensor (kgm2)) -> Inertia (kgm2)/1
  Forces And Moments simple model1/2(Moments) -> Moments (Nm)/1
  "transform to body axes "/1 -> Product/2
  Sum/1 -> Force (N)/1
  Forces And Moments simple model1/1(Forces) -> Sum/2
  Product/1 -> Sum/1
  Subsystem/1(Mass (Kg)) -> Product/1, Mass (Kg)/1
  DCMbe/1 -> "transform to body axes "/2, Subsystem/1(DCMbe)
  ulh (m)/1 -> "WGS84 Gravity Model  "/1
  "WGS84 Gravity Model  "/1 -> "transform to body axes "/1

== system testifintegratoriscorrect/Subsystem/If 0 after apogee1 ==
  In1 : Inport
  Clock1 : Clock
  Compare To Zero1 : simulink/Logic and Bit Operations/Compare To Zero  relop=<=  OutDataTypeStr=boolean
  Constant3 : Constant  Value=.5
  Logical Operator1 : Logic  AllPortsSameDT=off  OutDataTypeStr=boolean
  Relational Operator1 : RelationalOperator  Operator=>  OutDataTypeStr=boolean  RndMeth=Simplest
  Stop Simulation1 : Stop
  wires:
  Clock1/1 -> Relational Operator1/1
  Constant3/1 -> Relational Operator1/2
  In1/1 -> Compare To Zero1/1
  Logical Operator1/1 -> Stop Simulation1/1
  Compare To Zero1/1 -> Logical Operator1/2
  Relational Operator1/1 -> Logical Operator1/1

== system testifintegratoriscorrect/Subsystem/If 0 after apogee2 ==
  In1 : Inport
  Clock1 : Clock
  Compare To Zero1 : simulink/Logic and Bit Operations/Compare To Zero  relop=<=  OutDataTypeStr=boolean
  Constant3 : Constant  Value=.5
  Logical Operator1 : Logic  AllPortsSameDT=off  OutDataTypeStr=boolean
  Relational Operator1 : RelationalOperator  Operator=>  OutDataTypeStr=boolean  RndMeth=Simplest
  Stop Simulation1 : Stop
  wires:
  Clock1/1 -> Relational Operator1/1
  Constant3/1 -> Relational Operator1/2
  In1/1 -> Compare To Zero1/1
  Logical Operator1/1 -> Stop Simulation1/1
  Compare To Zero1/1 -> Logical Operator1/2
  Relational Operator1/1 -> Logical Operator1/1

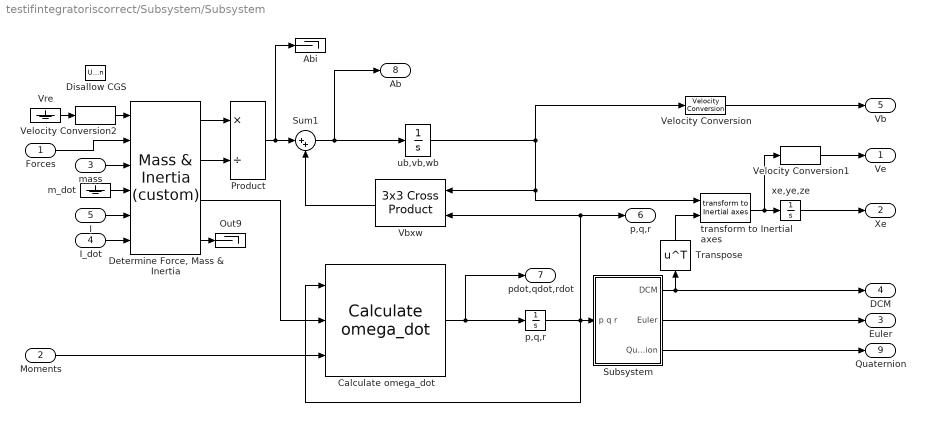
== system testifintegratoriscorrect/Subsystem/Subsystem ==
  Forces : Inport  Unit=N  PortDimensions=3
  Moments : Inport  Port=2  Unit=N*m  PortDimensions=3
  mass : Inport  Port=3  Unit=kg
  I_dot : Inport  Port=4  Unit=kg*m^2/s  PortDimensions=[3 3]
  I : Inport  Port=5  Unit=kg*m^2  PortDimensions=[3 3]
  Abi : Terminator
  Calculate omega_dot : shared6dofsys/Calculate omega_dot  aMode=aMode
      settings: SourceProductName=Aerospace Blockset  SourceProductBaseCode=AE
  "Determine Force, Mass & Inertia" : shared6dofsys/Mass & Inertia (custom)  aMode=aMode
      settings: SourceProductName=Aerospace Blockset  SourceProductBaseCode=AE
  Disallow CGS : UnitConfiguration  UnitSystemsStr=English,SI,SI (extended)  AllowAllUnitSystems=off
  Out9 : Terminator
  Product : Product  Inputs=*/  SaturateOnIntegerOverflow=on  OutDataTypeStr=Inherit: Same as first input
  Subsystem : Subsystem
  Sum1 : Sum  Inputs=|++  SaturateOnIntegerOverflow=on
  Transpose : Math  Operator=transpose  SaturateOnIntegerOverflow=on
  Vbxw : sharedutil/3x3 Cross Product  aMode=aMode
      settings: SourceProductBaseCode=AE
  Velocity Conversion : shared6dof/6DOF (Euler Angles)/Velocity Conversion  SystemSampleTime=-1
      settings: SourceProductName=Aerospace Blockset  SourceProductBaseCode=AE
  Velocity Conversion1 : shared6dof/6DOF (Euler Angles)/Velocity Conversion1  SystemSampleTime=-1
      settings: SourceProductName=Aerospace Blockset  SourceProductBaseCode=AE
  Velocity Conversion2 : shared6dof/6DOF (Euler Angles)/Velocity Conversion2  SystemSampleTime=-1
      settings: SourceProductName=Aerospace Blockset  SourceProductBaseCode=AE
  Vre : Ground
  m_dot : Ground
  "p,q,r " : Integrator  InitialCondition=[0 0 0]
  "transform to Inertial axes " : shared6dof/6DOF (Euler Angles)/transform to Inertial axes   SystemSampleTime=-1
      settings: SourceProductName=Aerospace Blockset  SourceProductBaseCode=AE
  ub,vb,wb : Integrator  InitialCondition=[0 0 0]
  xe,ye,ze : Integrator  InitialCondition=[0 0 0]
  Ve : Outport  Unit=m/s
  Xe : Outport  Port=2  Unit=m
  Euler : Outport  Port=3  Unit=rad
  DCM : Outport  Port=4  Unit=1
  Vb : Outport  Port=5  Unit=m/s
  p,q,r : Outport  Port=6  Unit=rad/s
  pdot,qdot,rdot : Outport  Port=7  Unit=rad/s^2
  Ab : Outport  Port=8  Unit=m/s^2
  Quaternion : Outport  Port=9
  wires:
  Subsystem/2(Euler) -> Euler/1
  "Determine Force, Mass & Inertia"/3 -> Calculate omega_dot/2
  "transform to Inertial axes "/1 -> xe,ye,ze/1, Velocity Conversion1/1
  ub,vb,wb/1 -> "transform to Inertial axes "/1, Vbxw/1, Velocity Conversion/1
  "p,q,r "/1 -> Subsystem/1(p q r), p,q,r/1, Vbxw/2, Calculate omega_dot/1
  Vbxw/1 -> Sum1/2
  xe,ye,ze/1 -> Xe/1
  mass/1 -> "Determine Force, Mass & Inertia"/3
  Velocity Conversion1/1 -> Ve/1
  Subsystem/1(DCM) -> DCM/1, Transpose/1
  Calculate omega_dot/1 -> pdot,qdot,rdot/1, "p,q,r "/1
  Transpose/1 -> "transform to Inertial axes "/2
  Sum1/1 -> ub,vb,wb/1, Ab/1
  Forces/1 -> "Determine Force, Mass & Inertia"/2
  "Determine Force, Mass & Inertia"/4 -> Out9/1
  I_dot/1 -> "Determine Force, Mass & Inertia"/6
  I/1 -> "Determine Force, Mass & Inertia"/5
  Velocity Conversion2/1 -> "Determine Force, Mass & Inertia"/1
  Product/1 -> Sum1/1, Abi/1
  Vre/1 -> Velocity Conversion2/1
  "Determine Force, Mass & Inertia"/1 -> Product/1
  "Determine Force, Mass & Inertia"/2 -> Product/2
  Velocity Conversion/1 -> Vb/1
  m_dot/1 -> "Determine Force, Mass & Inertia"/4
  Subsystem/3(Quaternion) -> Quaternion/1
  Moments/1 -> Calculate omega_dot/3

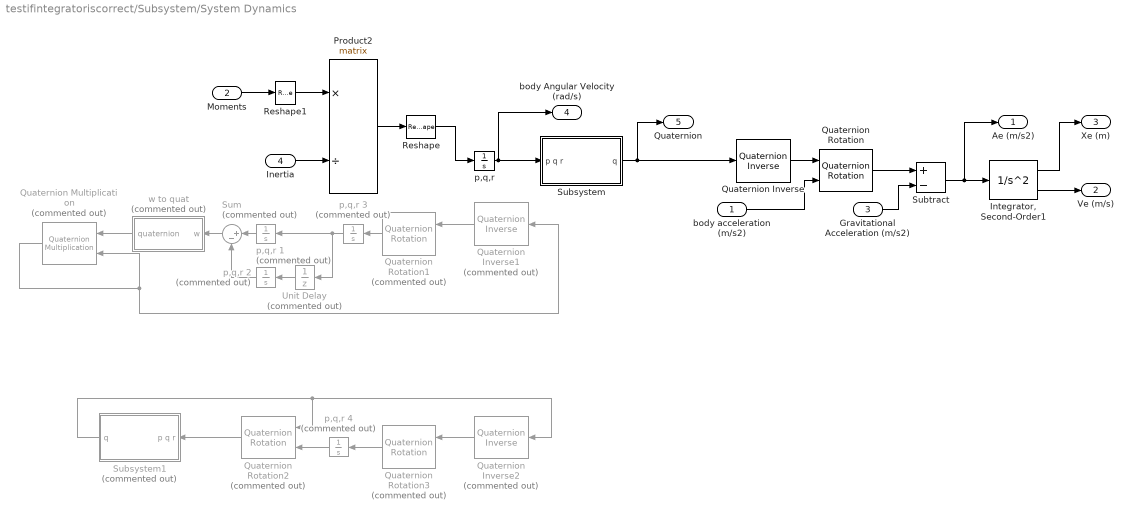
== system testifintegratoriscorrect/Subsystem/System Dynamics ==
  body acceleration (m/s2) : Inport
  Moments : Inport  Port=2
  Gravitational Acceleration (m/s2) : Inport  Port=3
  Inertia : Inport  Port=4
  "Integrator, Second-Order1" : SecondOrderIntegrator  ICX=0  LimitX=on  LowerLimitX=[-inf; -inf; 0]
  Product2 : Product  Inputs=*/  Multiplication=Matrix(*)  SaturateOnIntegerOverflow=on  OutDataTypeStr=Inherit: Same as first input
  Quaternion Inverse : aerolibutil/Quaternion Inverse
      settings: SourceProductName=Aerospace Blockset
  Quaternion Inverse1 : aerolibutil/Quaternion Inverse  Commented=on
      settings: SourceProductName=Aerospace Blockset
  Quaternion Inverse2 : aerolibutil/Quaternion Inverse  Commented=on
      settings: SourceProductName=Aerospace Blockset
  Quaternion Multiplication : aerolibutil/Quaternion Multiplication  Commented=on
  Quaternion Rotation : aerolibutil/Quaternion Rotation
  Quaternion Rotation1 : aerolibutil/Quaternion Rotation  Commented=on
  Quaternion Rotation2 : aerolibutil/Quaternion Rotation  Commented=on
  Quaternion Rotation3 : aerolibutil/Quaternion Rotation  Commented=on
  Reshape : Reshape
  Reshape1 : Reshape  OutputDimensionality=Row vector (2-D)
  Subsystem : Subsystem
  Subsystem1 : Subsystem  Commented=on
  Subtract : Sum  Inputs=+-
  Sum : Sum  Commented=on  Inputs=|+-
  Unit Delay : UnitDelay  Commented=on  SampleTime=-1  HasFrameUpgradeWarning=on
  "p,q,r " : Integrator
  p,q,r {1..4} (4 alike) : Integrator  Commented=on
  w to quat : MATLAB Function  Commented=on  TreatAsAtomicUnit=on
  Ae (m/s2) : Outport  Unit=m/s^2
  Ve (m/s) : Outport  Port=2  Unit=m/s
  Xe (m) : Outport  Port=3  Unit=m
  body Angular Velocity (rad/s) : Outport  Port=4  Unit=rad/s
  Quaternion : Outport  Port=5  Unit=1
  wires:
  body acceleration (m/s2)/1 -> Quaternion Rotation/2
  Subsystem/1(q) -> Quaternion/1, Quaternion Inverse/1
  Quaternion Inverse/1 -> Quaternion Rotation/1
  "Integrator, Second-Order1"/1 -> Xe (m)/1
  Gravitational Acceleration (m/s2)/1 -> Subtract/2
  Quaternion Rotation/1 -> Subtract/1
  "Integrator, Second-Order1"/2 -> Ve (m/s)/1
  Subtract/1 -> "Integrator, Second-Order1"/1, Ae (m/s2)/1
  Quaternion Inverse1/1 -> Quaternion Rotation1/1
  w to quat/1(quaternion) -> Quaternion Multiplication/1
  Unit Delay/1 -> p,q,r 2/1
  p,q,r 1/1 -> Sum/1
  p,q,r 2/1 -> Sum/2
  Sum/1 -> w to quat/1(w)
  p,q,r 3/1 -> Unit Delay/1, p,q,r 1/1
  Quaternion Rotation1/1 -> p,q,r 3/1
  Quaternion Rotation2/1 -> Subsystem1/1(p q r)
  Quaternion Multiplication/1 -> Quaternion Multiplication/2, Quaternion Inverse1/1
  Subsystem1/1(q) -> Quaternion Inverse2/1, Quaternion Rotation2/1
  Quaternion Rotation3/1 -> p,q,r 4/1
  Quaternion Inverse2/1 -> Quaternion Rotation3/1
  p,q,r 4/1 -> Quaternion Rotation2/2
  Inertia/1 -> Product2/2
  "p,q,r "/1 -> Subsystem/1(p q r), body Angular Velocity (rad/s)/1
  Product2/1 -> Reshape/1
  Reshape/1 -> "p,q,r "/1
  Reshape1/1 -> Product2/1
  Moments/1 -> Reshape1/1

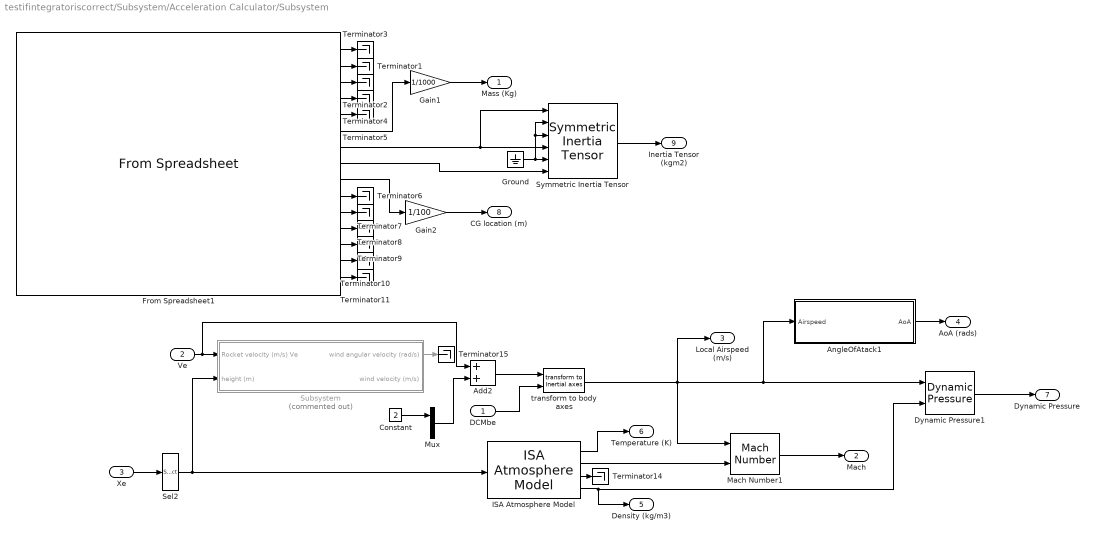
== system testifintegratoriscorrect/Subsystem/Acceleration Calculator/Subsystem ==
  DCMbe : Inport
  Ve : Inport  Port=2
  Xe : Inport  Port=3
  Add2 : Sum
  AngleOfAtack1 : MATLAB Function  TreatAsAtomicUnit=on
  Constant : Constant  Value=2
  Dynamic Pressure1 : aerolibasang/Dynamic Pressure
  From Spreadsheet1 : FromSpreadsheet  FileName=C:\Users\rag\Documents\GitHub\EPQ\OpenRocket\bodyacceleraiton.xlsx  SheetName=bodyacceleraiton  Range=A1:P4395  ExtrapolationBeforeFirstDataPoint=Hold first value  ExtrapolationAfterLastDataPoint=Hold last value
  Gain1 : Gain  Gain=1/1000
  Gain2 : Gain  Gain=1/100
  Ground : Ground
  ISA Atmosphere Model : aerolibatmos2/ISA Atmosphere Model  custom=on  g=9.80665  gamma=1.4  R=287.0531  L=0.0065  h_trop=11000  h_strat=20000  rho0=1.225  P0=Pressure  T0=Temperature  h0=0
      settings: SourceProductName=Aerospace Blockset
  Mach Number1 : aerolibasang/Mach Number
      settings: SourceProductName=Aerospace Blockset  SourceProductBaseCode=AE
  Mux : Mux  Inputs=3
  Sel2 : Selector  InputPortWidth=3  IndexOptions=Index vector (dialog)  Indices=3  OutputSizes=1
  Subsystem : Subsystem  Commented=on
  Symmetric Inertia Tensor : aerolibbdyn/Symmetric Inertia Tensor
      settings: SourceProductName=Aerospace Blockset  SourceProductBaseCode=AE
  Terminator{1..11,14..15} (13 alike) : Terminator
  "transform to body axes " : shared6dof/6DOF (Euler Angles)/transform to Inertial axes   SystemSampleTime=-1
      settings: SourceProductName=Aerospace Blockset  SourceProductBaseCode=AE
  Mass (Kg) : Outport
  Mach : Outport  Port=2
  Local Airspeed (m/s) : Outport  Port=3
  AoA (rads) : Outport  Port=4
  Density (kg/m3) : Outport  Port=5
  Temperature (K) : Outport  Port=6
  Dynamic Pressure : Outport  Port=7
  CG location (m) : Outport  Port=8
  Inertia Tensor (kgm2) : Outport  Port=9
  wires:
  From Spreadsheet1/8 -> Symmetric Inertia Tensor/6
  From Spreadsheet1/4 -> Terminator4/1
  "transform to body axes "/1 -> Local Airspeed (m/s)/1, AngleOfAtack1/1(Airspeed), Dynamic Pressure1/1, Mach Number1/1
  ISA Atmosphere Model/4 -> Density (kg/m3)/1, Dynamic Pressure1/2
  From Spreadsheet1/5 -> Terminator5/1
  From Spreadsheet1/9 -> Gain2/1
  From Spreadsheet1/6 -> Gain1/1
  ISA Atmosphere Model/2 -> Mach Number1/2
  ISA Atmosphere Model/1 -> Temperature (K)/1
  Dynamic Pressure1/1 -> Dynamic Pressure/1
  Mach Number1/1 -> Mach/1
  From Spreadsheet1/12 -> Terminator8/1
  AngleOfAtack1/1(AoA) -> AoA (rads)/1
  ISA Atmosphere Model/3 -> Terminator14/1
  Gain2/1 -> CG location (m)/1
  From Spreadsheet1/7 -> Symmetric Inertia Tensor/1, Symmetric Inertia Tensor/4
  From Spreadsheet1/11 -> Terminator7/1
  Xe/1 -> Sel2/1
  From Spreadsheet1/3 -> Terminator2/1
  From Spreadsheet1/14 -> Terminator10/1
  From Spreadsheet1/2 -> Terminator1/1
  From Spreadsheet1/1 -> Terminator3/1
  From Spreadsheet1/13 -> Terminator9/1
  From Spreadsheet1/15 -> Terminator11/1
  Gain1/1 -> Mass (Kg)/1
  Ground/1 -> Symmetric Inertia Tensor/2, Symmetric Inertia Tensor/3, Symmetric Inertia Tensor/5
  Symmetric Inertia Tensor/1 -> Inertia Tensor (kgm2)/1
  From Spreadsheet1/10 -> Terminator6/1
  Subsystem/1(wind angular velocity (rad/s)) -> Terminator15/1
  Ve/1 -> Subsystem/1(Rocket velocity (m/s) Ve), Add2/1
  Sel2/1 -> Subsystem/2(height (m)), ISA Atmosphere Model/1
  Constant/1 -> Mux/1
  Mux/1 -> Add2/2
  Add2/1 -> "transform to body axes "/1
  DCMbe/1 -> "transform to body axes "/2

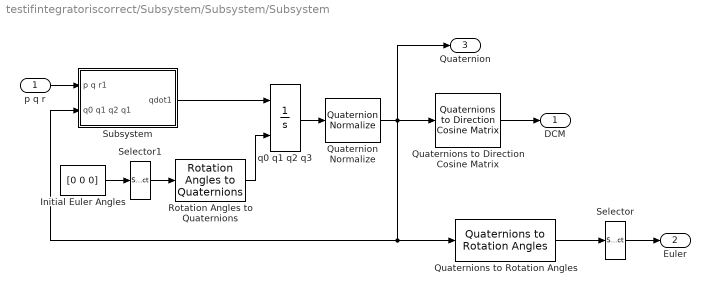
== system testifintegratoriscorrect/Subsystem/Subsystem/Subsystem ==
  p q r : Inport
  Initial Euler Angles : Constant  Value=[0 0 0]
  Quaternion Normalize : sharedutil/Quaternion Normalize  aMode=aMode
      settings: SourceProductName=Aerospace Blockset  SourceProductBaseCode=AE
  Quaternions to Direction Cosine Matrix : sharedtransform/Quaternions to  Direction Cosine Matrix  aMode=aMode
      settings: SourceProductName=Aerospace Blockset  SourceProductBaseCode=AE
  Quaternions to Rotation Angles : sharedtransform/Quaternions to Rotation Angles  rotationOrder=ZYX  aMode=aMode
      settings: SourceProductBaseCode=AE
  Rotation Angles to Quaternions : sharedtransform/Rotation Angles to Quaternions  rotationOrder=ZYX  aMode=aMode
      settings: SourceProductName=Aerospace Blockset  SourceProductBaseCode=AE
  Selector : Selector  InputPortWidth=3  IndexOptions=Index vector (dialog)  Indices=[3 2 1]  OutputSizes=1
  Selector1 : Selector  InputPortWidth=3  IndexOptions=Index vector (dialog)  Indices=[3 2 1]  OutputSizes=1
  Subsystem : Subsystem
  q0 q1 q2 q3 : Integrator  InitialConditionSource=external  InitialCondition=[e0_0 e1_0 e2_0 e3_0]
  DCM : Outport
  Euler : Outport  Port=2
  Quaternion : Outport  Port=3
  wires:
  Rotation Angles to Quaternions/1 -> q0 q1 q2 q3/2
  Selector/1 -> Euler/1
  Initial Euler Angles/1 -> Selector1/1
  Selector1/1 -> Rotation Angles to Quaternions/1
  q0 q1 q2 q3/1 -> Quaternion Normalize/1
  Quaternions to Direction Cosine Matrix/1 -> DCM/1
  Subsystem/1(qdot1) -> q0 q1 q2 q3/1
  p q r/1 -> Subsystem/1(p q r1)
  Quaternions to Rotation Angles/1 -> Selector/1
  Quaternion Normalize/1 -> Quaternion/1, Subsystem/2(q0 q1 q2 q1), Quaternions to Rotation Angles/1, Quaternions to Direction Cosine Matrix/1

== system testifintegratoriscorrect/Subsystem/System Dynamics/Subsystem ==
  p q r : Inport
  Initial Euler Angles : Constant  Value=[0 0 0]
  Rotation Angles to Quaternions : sharedtransform/Rotation Angles to Quaternions  rotationOrder=ZYX  aMode=aMode
      settings: SourceProductName=Aerospace Blockset  SourceProductBaseCode=AE
  Selector1 : Selector  InputPortWidth=3  IndexOptions=Index vector (dialog)  Indices=[3 2 1]  OutputSizes=1
  Subsystem : Subsystem
  q0 q1 q2 q3 : Integrator  InitialConditionSource=external  InitialCondition=[e0_0 e1_0 e2_0 e3_0]
  q : Outport
  wires:
  Rotation Angles to Quaternions/1 -> q0 q1 q2 q3/2
  Initial Euler Angles/1 -> Selector1/1
  Subsystem/1(qdot2) -> q0 q1 q2 q3/1
  Selector1/1 -> Rotation Angles to Quaternions/1
  p q r/1 -> Subsystem/1(p q r1)
  q0 q1 q2 q3/1 -> Subsystem/2(q0 q1 q2 q1), q/1

== system testifintegratoriscorrect/Subsystem/System Dynamics/Subsystem1 ==
  p q r : Inport
  Initial Euler Angles : Constant  Value=[0 0 0]
  Quaternion Normalize : sharedutil/Quaternion Normalize  aMode=aMode
      settings: SourceProductName=Aerospace Blockset  SourceProductBaseCode=AE
  Rotation Angles to Quaternions : sharedtransform/Rotation Angles to Quaternions  rotationOrder=ZYX  aMode=aMode
      settings: SourceProductName=Aerospace Blockset  SourceProductBaseCode=AE
  Selector1 : Selector  InputPortWidth=3  IndexOptions=Index vector (dialog)  Indices=[3 2 1]  OutputSizes=1
  Subsystem : Subsystem
  q0 q1 q2 q3 : Integrator  InitialConditionSource=external  InitialCondition=[e0_0 e1_0 e2_0 e3_0]
  q : Outport
  wires:
  Rotation Angles to Quaternions/1 -> q0 q1 q2 q3/2
  Initial Euler Angles/1 -> Selector1/1
  Subsystem/1(qdot2) -> q0 q1 q2 q3/1
  Selector1/1 -> Rotation Angles to Quaternions/1
  p q r/1 -> Subsystem/1(p q r1)
  q0 q1 q2 q3/1 -> Quaternion Normalize/1, Subsystem/2(q0 q1 q2 q1)
  Quaternion Normalize/1 -> q/1

== system testifintegratoriscorrect/Subsystem/Acceleration Calculator/Subsystem/Subsystem ==
  Rocket velocity (m/s) Ve : Inport
  height (m) : Inport  Port=2
  DCM : MATLAB Function  TreatAsAtomicUnit=on
  Discrete Wind Gust Model : aerolibwind2/Discrete Wind Gust Model  units=Metric (MKS)  Gx=on  Gy=on  Gz=on  t_0=GustStart  d_m=GustLength  v_m=GuestAmplitude
      settings: SourceProductName=Aerospace Blockset
  MATLAB Function : MATLAB Function  TreatAsAtomicUnit=on
  Sum : Sum  Inputs=3
  Von Karman Wind Turbulence Model (Continuous (+q +r)) : aerolibwind2/Dryden Wind Turbulence Model  (Continuous (+q -r))  units=Metric (MKS)  spec=MIL-F-8785C  model=Discrete Dryden (+q -r)  W20=ShearSpeed  Wdeg=ShearDirection  TurbProb=10^-2 - Light  L_high=762  Wingspan=10  ts=0.1  Seed=[23341 23342 23343 23344]  T_on=on
      settings: SourceProductName=Aerospace Blockset
  Wind Shear Model : aerolibwind2/Wind Shear Model  units=Metric (MKS)  phase=Category C - Terminal Flight Phase  W_20=ShearSpeed  Wdeg=ShearDirection
      settings: SourceProductName=Aerospace Blockset
  wind angular velocity (rad/s) : Outport
  wind velocity (m/s) : Outport  Port=2
  wires:
  height (m)/1 -> Wind Shear Model/1, Von Karman Wind Turbulence Model (Continuous (+q +r))/1
  Discrete Wind Gust Model/1 -> Sum/1
  DCM/1(DCM) -> Von Karman Wind Turbulence Model (Continuous (+q +r))/3, Wind Shear Model/2
  MATLAB Function/1(magnitude) -> Von Karman Wind Turbulence Model (Continuous (+q +r))/2, Discrete Wind Gust Model/1
  Sum/1 -> wind velocity (m/s)/1
  Wind Shear Model/1 -> Sum/3
  Von Karman Wind Turbulence Model (Continuous (+q +r))/1 -> Sum/2
  Von Karman Wind Turbulence Model (Continuous (+q +r))/2 -> wind angular velocity (rad/s)/1
  Rocket velocity (m/s) Ve/1 -> MATLAB Function/1(u)
